simulink model "uncontroled"  (R2021a)
settings: Solver=FixedStepAuto  StartTime=start_time  StopTime=stop_time  FixedStep=min_step  MinStep=min_step  RelTol=1e-3
values from neighbouring files (symbols this model uses):
  amp = 2000    [controlprj.m]
  c = 0    [controlprj.m]
  delta_t = 0.001    [controlprj.m]
  g = 9.80665    [controlprj.m]
  initial_disp = 0.01    [controlprj.m]
  initial_velocity = 0.1    [controlprj.m]
  k = 29127    [controlprj.m]
  m = 5873    [controlprj.m]
  switchF = 1    [controlprj.m]
  target_t = 30    [controlprj.m]
libraries: simulink x1
settings Model: Creator=mehrab  LastModifiedBy=mehrab
settings SolverCC: AlgebraicLoopSolver=TrustRegion
settings DataIOCC: SaveFormat=StructureWithTime  ReturnWorkspaceOutputs=off
settings OptimizationCC: LifeSpan=inf
settings DebuggingCC: SFExecutionAtInitializationDiag=none  SFMachineParentedDataDiag=warning  ArithmeticOperatorsInVariantConditions=warning
settings HardwareCC: ProdBitPerSizeT=32  ProdBitPerPtrDiffT=32  ProdWordSize=32  ProdHWDeviceType=Specified
settings SFSimCC: SimUseLocalCustomCode=off  CustomCodeUndefinedFunction=UseInterfaceOnly
settings RTWCC: RTWUseLocalCustomCode=off
settings CodeAppCC: StateflowObjectComments=on

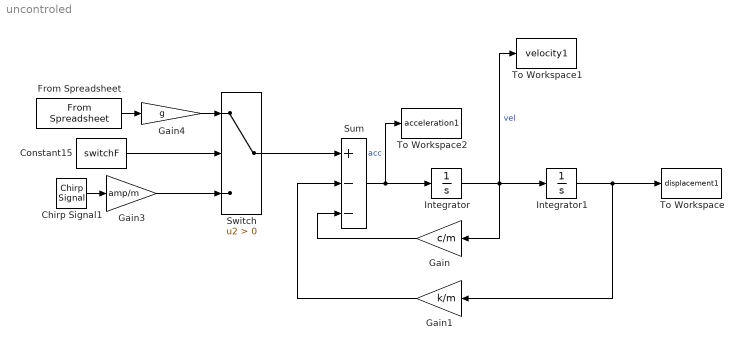
== system uncontroled ==
  Chirp Signal1 : simulink/Sources/Chirp Signal  f1=initial_freq  T=target_t  f2=freq_target
  Constant15 : Constant  Value=switchF
  From Spreadsheet : FromSpreadsheet  FileName=elcentro.xlsx
  Gain : Gain  Gain=c/m
  Gain1 : Gain  Gain=k/m
  Gain3 : Gain  Gain=amp/m
  Gain4 : Gain  Gain=g
  Integrator : Integrator  InitialCondition=initial_velocity
  Integrator1 : Integrator  InitialCondition=initial_disp
  Sum : Sum  Inputs=+--
  Switch : Switch  Criteria=u2 > Threshold
  To Workspace : ToWorkspace  VariableName=displacement1  SampleTime=delta_t
  To Workspace1 : ToWorkspace  VariableName=velocity1  SampleTime=delta_t
  To Workspace2 : ToWorkspace  VariableName=acceleration1  SampleTime=delta_t
  wires:
  Sum/1 -> To Workspace2/1, Integrator/1  "acc"
  Integrator/1 -> To Workspace1/1, Gain/1, Integrator1/1  "vel"
  Gain/1 -> Sum/3
  Integrator1/1 -> Gain1/1, To Workspace/1
  Gain1/1 -> Sum/2
  Constant15/1 -> Switch/2
  Gain3/1 -> Switch/3
  Chirp Signal1/1 -> Gain3/1
  Switch/1 -> Sum/1
  From Spreadsheet/1 -> Gain4/1
  Gain4/1 -> Switch/1
